simulink model "case3"  (R2024b)
settings: Solver=FixedStepAuto  StartTime=0  StopTime=1  FixedStep=1e-7  RelTol=1e-3
values from neighbouring files (symbols this model uses):
  SG_D_1_D = 0.01056    [IEEE9_case_parameters.m]    (also in case1_parameters.m; case2_parameters.m; case3_parameters.m; case4_parameters.m)
  SG_D_1_EnableSaturation = 0    [IEEE9_case_parameters.m]    (also in case1_parameters.m; case2_parameters.m; case3_parameters.m; case4_parameters.m)
  SG_D_1_f0 = 60    [IEEE9_case_parameters.m]    (also in case1_parameters.m; case2_parameters.m; case3_parameters.m; case4_parameters.m)
  SG_D_1_H = 7.5    [IEEE9_case_parameters.m]    (also in case1_parameters.m; case2_parameters.m; case3_parameters.m; case4_parameters.m)
  SG_D_1_K_A = 20    [IEEE9_case_parameters.m]    (also in case1_parameters.m; case2_parameters.m; case3_parameters.m; case4_parameters.m)
  SG_D_1_K_E = 1.000000e+1    (= 10)    [IEEE9_case_parameters.m]    (also in case1_parameters.m; case2_parameters.m; case3_parameters.m; case4_parameters.m)
  SG_D_1_K_F = 2.363    [IEEE9_case_parameters.m]    (also in case1_parameters.m; case2_parameters.m; case3_parameters.m; case4_parameters.m)
  SG_D_1_K_s = 0.5    [IEEE9_case_parameters.m]    (also in case1_parameters.m = 5; case2_parameters.m = 5; case3_parameters.m = 5; case4_parameters.m = 5)
  SG_D_1_R_a = 0.001088    [IEEE9_case_parameters.m]    (also in case1_parameters.m; case2_parameters.m; case3_parameters.m; case4_parameters.m)
  SG_D_1_S_A = 1    [IEEE9_case_parameters.m]    (also in case1_parameters.m; case2_parameters.m; case3_parameters.m; case4_parameters.m)
  SG_D_1_S_B = 0.103    [IEEE9_case_parameters.m]    (also in case1_parameters.m; case2_parameters.m; case3_parameters.m; case4_parameters.m)
  SG_D_1_S_N = 10.659857    [IEEE9_case_parameters.m]    (also in case1_parameters.m; case2_parameters.m; case3_parameters.m; case4_parameters.m)
  SG_D_1_SpeedPara = 200    [IEEE9_case_parameters.m]    (also in case1_parameters.m; case2_parameters.m; case3_parameters.m; case4_parameters.m)
  SG_D_1_T_0 = 0.720173    [IEEE9_case_parameters.m]    (also in case1_parameters.m = 0.755522; case2_parameters.m = 0.808931; case3_parameters.m = 0.869402; case4_parameters.m = 0.729316)
  SG_D_1_T_1 = 0.3    [IEEE9_case_parameters.m]    (also in case1_parameters.m; case2_parameters.m; case3_parameters.m; case4_parameters.m)
  SG_D_1_T_2 = 0.05    [IEEE9_case_parameters.m]    (also in case1_parameters.m; case2_parameters.m; case3_parameters.m; case4_parameters.m)
  SG_D_1_T_3 = 0.02    [IEEE9_case_parameters.m]    (also in case1_parameters.m; case2_parameters.m; case3_parameters.m; case4_parameters.m)
  SG_D_1_T_4 = 0.005    [IEEE9_case_parameters.m]    (also in case1_parameters.m; case2_parameters.m; case3_parameters.m; case4_parameters.m)
  SG_D_1_T_A = 0.02    [IEEE9_case_parameters.m]    (also in case1_parameters.m; case2_parameters.m; case3_parameters.m; case4_parameters.m)
  SG_D_1_T_dd = 8.000000e+0    (= 8)    [IEEE9_case_parameters.m]    (also in case1_parameters.m; case2_parameters.m; case3_parameters.m; case4_parameters.m)
  SG_D_1_T_ddd = 0.04    [IEEE9_case_parameters.m]    (also in case1_parameters.m; case2_parameters.m; case3_parameters.m; case4_parameters.m)
  SG_D_1_T_E = 0.314    [IEEE9_case_parameters.m]    (also in case1_parameters.m; case2_parameters.m; case3_parameters.m; case4_parameters.m)
  SG_D_1_T_F = 0.35    [IEEE9_case_parameters.m]    (also in case1_parameters.m; case2_parameters.m; case3_parameters.m; case4_parameters.m)
  SG_D_1_T_qd = 0.8    [IEEE9_case_parameters.m]    (also in case1_parameters.m; case2_parameters.m; case3_parameters.m; case4_parameters.m)
  SG_D_1_T_qdd = 0.02    [IEEE9_case_parameters.m]    (also in case1_parameters.m; case2_parameters.m; case3_parameters.m; case4_parameters.m)
  SG_D_1_T_speed = 0.1    [IEEE9_case_parameters.m]    (also in case1_parameters.m = 200; case2_parameters.m = 200; case3_parameters.m = 200; case4_parameters.m = 200)
  SG_D_1_T_w = 0.5    [IEEE9_case_parameters.m]    (also in case1_parameters.m; case2_parameters.m; case3_parameters.m; case4_parameters.m)
  SG_D_1_V_ref = 1.990276    [IEEE9_case_parameters.m]    (also in case1_parameters.m = 2.042296; case2_parameters.m = 2.051388; case3_parameters.m = 2.089584; case4_parameters.m = 2.01845)
  SG_D_1_w_ref = 376.991118    [IEEE9_case_parameters.m]    (also in case1_parameters.m; case2_parameters.m; case3_parameters.m; case4_parameters.m)
  SG_D_1_wb = 6.000000e+1    (= 60)    [IEEE9_case_parameters.m]    (also in case1_parameters.m; case2_parameters.m; case3_parameters.m; case4_parameters.m)
  SG_D_1_x_d = 1.9    [IEEE9_case_parameters.m]    (also in case1_parameters.m; case2_parameters.m; case3_parameters.m; case4_parameters.m)
  SG_D_1_x_dd = 0.302    [IEEE9_case_parameters.m]    (also in case1_parameters.m; case2_parameters.m; case3_parameters.m; case4_parameters.m)
  SG_D_1_x_ddd = 0.204    [IEEE9_case_parameters.m]    (also in case1_parameters.m; case2_parameters.m; case3_parameters.m; case4_parameters.m)
  SG_D_1_x_l = 0.05    [IEEE9_case_parameters.m]    (also in case1_parameters.m; case2_parameters.m; case3_parameters.m; case4_parameters.m)
  SG_D_1_x_q = 1.3    [IEEE9_case_parameters.m]    (also in case1_parameters.m; case2_parameters.m; case3_parameters.m; case4_parameters.m)
  SG_D_1_x_qd = 0.5    [IEEE9_case_parameters.m]    (also in case1_parameters.m; case2_parameters.m; case3_parameters.m; case4_parameters.m)
  SG_D_1_x_qdd = 0.3    [IEEE9_case_parameters.m]    (also in case1_parameters.m; case2_parameters.m; case3_parameters.m; case4_parameters.m)
  SG_D_2_D = 0.02    [IEEE9_case_parameters.m]    (also in case1_parameters.m; case2_parameters.m; case3_parameters.m; case4_parameters.m)
  SG_D_2_EnableSaturation = 0    [IEEE9_case_parameters.m]    (also in case1_parameters.m; case2_parameters.m; case3_parameters.m; case4_parameters.m)
  SG_D_2_f0 = 60    [IEEE9_case_parameters.m]    (also in case1_parameters.m; case2_parameters.m; case3_parameters.m; case4_parameters.m)
  SG_D_2_H = 8.000000e+0    (= 8)    [IEEE9_case_parameters.m]    (also in case1_parameters.m; case2_parameters.m; case3_parameters.m; case4_parameters.m)
  SG_D_2_K_A = 20    [IEEE9_case_parameters.m]    (also in case1_parameters.m; case2_parameters.m; case3_parameters.m; case4_parameters.m)
  SG_D_2_K_E = 1.000000e+1    (= 10)    [IEEE9_case_parameters.m]    (also in case1_parameters.m; case2_parameters.m; case3_parameters.m; case4_parameters.m)
  SG_D_2_K_F = 2.363    [IEEE9_case_parameters.m]    (also in case1_parameters.m; case2_parameters.m; case3_parameters.m; case4_parameters.m)
  SG_D_2_K_s = 0.5    [IEEE9_case_parameters.m]    (also in case1_parameters.m = 4; case2_parameters.m = 4; case3_parameters.m = 4; case4_parameters.m = 4)
  SG_D_2_R_a = 0.001088    [IEEE9_case_parameters.m]    (also in case1_parameters.m; case2_parameters.m; case3_parameters.m; case4_parameters.m)
  SG_D_2_S_A = 1    [IEEE9_case_parameters.m]    (also in case1_parameters.m; case2_parameters.m; case3_parameters.m; case4_parameters.m)
  SG_D_2_S_B = 0.103    [IEEE9_case_parameters.m]    (also in case1_parameters.m; case2_parameters.m; case3_parameters.m; case4_parameters.m)
  SG_D_2_S_N = 10.659857    [IEEE9_case_parameters.m]    (also in case1_parameters.m; case2_parameters.m; case3_parameters.m; case4_parameters.m)
  SG_D_2_SpeedPara = 200    [IEEE9_case_parameters.m]    (also in case1_parameters.m; case2_parameters.m; case3_parameters.m; case4_parameters.m)
  SG_D_2_T_0 = 1.632913    [IEEE9_case_parameters.m]    (also in case1_parameters.m = 1.632925; case2_parameters.m = 1.632915; case3_parameters.m = 1.632914; case4_parameters.m = 1.632927)
  SG_D_2_T_1 = 0.2    [IEEE9_case_parameters.m]    (also in case1_parameters.m; case2_parameters.m; case3_parameters.m; case4_parameters.m)
  SG_D_2_T_2 = 0.05    [IEEE9_case_parameters.m]    (also in case1_parameters.m; case2_parameters.m; case3_parameters.m; case4_parameters.m)
  SG_D_2_T_3 = 0.02    [IEEE9_case_parameters.m]    (also in case1_parameters.m; case2_parameters.m; case3_parameters.m; case4_parameters.m)
  SG_D_2_T_4 = 0.005    [IEEE9_case_parameters.m]    (also in case1_parameters.m; case2_parameters.m; case3_parameters.m; case4_parameters.m)
  SG_D_2_T_A = 0.02    [IEEE9_case_parameters.m]    (also in case1_parameters.m; case2_parameters.m; case3_parameters.m; case4_parameters.m)
  SG_D_2_T_dd = 7.9    [IEEE9_case_parameters.m]    (also in case1_parameters.m; case2_parameters.m; case3_parameters.m; case4_parameters.m)
  SG_D_2_T_ddd = 0.04    [IEEE9_case_parameters.m]    (also in case1_parameters.m; case2_parameters.m; case3_parameters.m; case4_parameters.m)
  SG_D_2_T_E = 0.314    [IEEE9_case_parameters.m]    (also in case1_parameters.m; case2_parameters.m; case3_parameters.m; case4_parameters.m)
  SG_D_2_T_F = 0.35    [IEEE9_case_parameters.m]    (also in case1_parameters.m; case2_parameters.m; case3_parameters.m; case4_parameters.m)
  SG_D_2_T_qd = 0.8    [IEEE9_case_parameters.m]    (also in case1_parameters.m; case2_parameters.m; case3_parameters.m; case4_parameters.m)
  SG_D_2_T_qdd = 0.015    [IEEE9_case_parameters.m]    (also in case1_parameters.m; case2_parameters.m; case3_parameters.m; case4_parameters.m)
  SG_D_2_T_speed = 0.1    [IEEE9_case_parameters.m]    (also in case1_parameters.m = 150; case2_parameters.m = 150; case3_parameters.m = 150; case4_parameters.m = 150)
  SG_D_2_T_w = 0.35    [IEEE9_case_parameters.m]    (also in case1_parameters.m; case2_parameters.m; case3_parameters.m; case4_parameters.m)
  SG_D_2_V_ref = 2.58547    [IEEE9_case_parameters.m]    (also in case1_parameters.m = 2.597896; case2_parameters.m = 2.587136; case3_parameters.m = 2.586042; case4_parameters.m = 2.599679)
  SG_D_2_w_ref = 376.991118    [IEEE9_case_parameters.m]    (also in case1_parameters.m; case2_parameters.m; case3_parameters.m; case4_parameters.m)
  SG_D_2_wb = 6.000000e+1    (= 60)    [IEEE9_case_parameters.m]    (also in case1_parameters.m; case2_parameters.m; case3_parameters.m; case4_parameters.m)
  SG_D_2_x_d = 1.8    [IEEE9_case_parameters.m]    (also in case1_parameters.m; case2_parameters.m; case3_parameters.m; case4_parameters.m)
  SG_D_2_x_dd = 0.302    [IEEE9_case_parameters.m]    (also in case1_parameters.m; case2_parameters.m; case3_parameters.m; case4_parameters.m)
  SG_D_2_x_ddd = 0.204    [IEEE9_case_parameters.m]    (also in case1_parameters.m; case2_parameters.m; case3_parameters.m; case4_parameters.m)
  SG_D_2_x_l = 0.05    [IEEE9_case_parameters.m]    (also in case1_parameters.m; case2_parameters.m; case3_parameters.m; case4_parameters.m)
  SG_D_2_x_q = 1.25    [IEEE9_case_parameters.m]    (also in case1_parameters.m; case2_parameters.m; case3_parameters.m; case4_parameters.m)
  SG_D_2_x_qd = 0.5    [IEEE9_case_parameters.m]    (also in case1_parameters.m; case2_parameters.m; case3_parameters.m; case4_parameters.m)
  SG_D_2_x_qdd = 0.3    [IEEE9_case_parameters.m]    (also in case1_parameters.m; case2_parameters.m; case3_parameters.m; case4_parameters.m)
  SG_D_3_D = 0.02    [IEEE9_case_parameters.m]    (also in case1_parameters.m; case2_parameters.m; case3_parameters.m; case4_parameters.m)
  SG_D_3_EnableSaturation = 0    [IEEE9_case_parameters.m]    (also in case1_parameters.m; case2_parameters.m; case3_parameters.m; case4_parameters.m)
  SG_D_3_f0 = 60    [IEEE9_case_parameters.m]    (also in case1_parameters.m; case2_parameters.m; case3_parameters.m; case4_parameters.m)
  SG_D_3_H = 7.7    [IEEE9_case_parameters.m]    (also in case1_parameters.m; case2_parameters.m; case3_parameters.m; case4_parameters.m)
  SG_D_3_K_A = 20    [IEEE9_case_parameters.m]    (also in case1_parameters.m; case2_parameters.m; case3_parameters.m; case4_parameters.m)
  SG_D_3_K_E = 1.000000e+1    (= 10)    [IEEE9_case_parameters.m]    (also in case1_parameters.m; case2_parameters.m; case3_parameters.m; case4_parameters.m)
  SG_D_3_K_F = 2.363    [IEEE9_case_parameters.m]    (also in case1_parameters.m; case2_parameters.m; case3_parameters.m; case4_parameters.m)
  SG_D_3_K_s = 0.2    [IEEE9_case_parameters.m]    (also in case1_parameters.m = 2; case2_parameters.m = 2; case3_parameters.m = 2; case4_parameters.m = 2)
  SG_D_3_R_a = 0.001088    [IEEE9_case_parameters.m]    (also in case1_parameters.m; case2_parameters.m; case3_parameters.m; case4_parameters.m)
  SG_D_3_S_A = 1    [IEEE9_case_parameters.m]    (also in case1_parameters.m; case2_parameters.m; case3_parameters.m; case4_parameters.m)
  SG_D_3_S_B = 0.103    [IEEE9_case_parameters.m]    (also in case1_parameters.m; case2_parameters.m; case3_parameters.m; case4_parameters.m)
  SG_D_3_S_N = 10.659857    [IEEE9_case_parameters.m]    (also in case1_parameters.m; case2_parameters.m; case3_parameters.m; case4_parameters.m)
  SG_D_3_SpeedPara = 200    [IEEE9_case_parameters.m]    (also in case1_parameters.m; case2_parameters.m; case3_parameters.m; case4_parameters.m)
  SG_D_3_T_0 = 0.850788    [IEEE9_case_parameters.m]    (also in case1_parameters.m = 0.850786; case2_parameters.m = 0.850787; case3_parameters.m; case4_parameters.m = 0.850786)
  SG_D_3_T_1 = 0.2    [IEEE9_case_parameters.m]    (also in case1_parameters.m; case2_parameters.m; case3_parameters.m; case4_parameters.m)
  SG_D_3_T_2 = 0.05    [IEEE9_case_parameters.m]    (also in case1_parameters.m; case2_parameters.m; case3_parameters.m; case4_parameters.m)
  SG_D_3_T_3 = 0.02    [IEEE9_case_parameters.m]    (also in case1_parameters.m; case2_parameters.m; case3_parameters.m; case4_parameters.m)
  SG_D_3_T_4 = 0.005    [IEEE9_case_parameters.m]    (also in case1_parameters.m; case2_parameters.m; case3_parameters.m; case4_parameters.m)
  SG_D_3_T_A = 0.02    [IEEE9_case_parameters.m]    (also in case1_parameters.m; case2_parameters.m; case3_parameters.m; case4_parameters.m)
  SG_D_3_T_dd = 8.1    [IEEE9_case_parameters.m]    (also in case1_parameters.m; case2_parameters.m; case3_parameters.m; case4_parameters.m)
  SG_D_3_T_ddd = 0.04    [IEEE9_case_parameters.m]    (also in case1_parameters.m; case2_parameters.m; case3_parameters.m; case4_parameters.m)
  SG_D_3_T_E = 0.314    [IEEE9_case_parameters.m]    (also in case1_parameters.m; case2_parameters.m; case3_parameters.m; case4_parameters.m)
  SG_D_3_T_F = 0.35    [IEEE9_case_parameters.m]    (also in case1_parameters.m; case2_parameters.m; case3_parameters.m; case4_parameters.m)
  SG_D_3_T_qd = 0.8    [IEEE9_case_parameters.m]    (also in case1_parameters.m; case2_parameters.m; case3_parameters.m; case4_parameters.m)
  SG_D_3_T_qdd = 0.015    [IEEE9_case_parameters.m]    (also in case1_parameters.m; case2_parameters.m; case3_parameters.m; case4_parameters.m)
  SG_D_3_T_speed = 0.1    [IEEE9_case_parameters.m]    (also in case1_parameters.m = 180; case2_parameters.m = 180; case3_parameters.m = 180; case4_parameters.m = 180)
  SG_D_3_T_w = 0.4    [IEEE9_case_parameters.m]    (also in case1_parameters.m; case2_parameters.m; case3_parameters.m; case4_parameters.m)
  SG_D_3_V_ref = 1.892727    [IEEE9_case_parameters.m]    (also in case1_parameters.m = 1.906439; case2_parameters.m = 1.895535; case3_parameters.m = 1.892105; case4_parameters.m = 1.906598)
  SG_D_3_w_ref = 376.991118    [IEEE9_case_parameters.m]    (also in case1_parameters.m; case2_parameters.m; case3_parameters.m; case4_parameters.m)
  SG_D_3_wb = 6.000000e+1    (= 60)    [IEEE9_case_parameters.m]    (also in case1_parameters.m; case2_parameters.m; case3_parameters.m; case4_parameters.m)
  SG_D_3_x_d = 1.85    [IEEE9_case_parameters.m]    (also in case1_parameters.m; case2_parameters.m; case3_parameters.m; case4_parameters.m)
  SG_D_3_x_dd = 0.302    [IEEE9_case_parameters.m]    (also in case1_parameters.m; case2_parameters.m; case3_parameters.m; case4_parameters.m)
  SG_D_3_x_ddd = 0.204    [IEEE9_case_parameters.m]    (also in case1_parameters.m; case2_parameters.m; case3_parameters.m; case4_parameters.m)
  SG_D_3_x_l = 0.05    [IEEE9_case_parameters.m]    (also in case1_parameters.m; case2_parameters.m; case3_parameters.m; case4_parameters.m)
  SG_D_3_x_q = 1.2    [IEEE9_case_parameters.m]    (also in case1_parameters.m; case2_parameters.m; case3_parameters.m; case4_parameters.m)
  SG_D_3_x_qd = 0.5    [IEEE9_case_parameters.m]    (also in case1_parameters.m; case2_parameters.m; case3_parameters.m; case4_parameters.m)
  SG_D_3_x_qdd = 0.3    [IEEE9_case_parameters.m]    (also in case1_parameters.m; case2_parameters.m; case3_parameters.m; case4_parameters.m)
(part 6 of 12)

== system case3/SG_D_1/d_psi_kq_SG_D_1_block ==
  note: d_psi_kq_SG_D_1 in case3
      | $-\frac{\psi _{\mathrm{gq},\mathrm{SG},D,1}+\psi _{\mathrm{kq},\mathrm{SG},D,1}+\frac{\left(x_{l}-x_{\mathrm{qd}}\right)\,\left(\psi _{q,\mathrm{SG},D,1}+\frac{\psi _{\mathrm{gq},\mathrm{SG},D,1}\,\left(x_{l}-x_{\mathrm{qdd}}\right)}{x_{l}-x_{\mathrm{qd}}}+\frac{\psi _{\mathrm{kq},\mathrm{SG},D,1}\,\left(x_{\mathrm{qd}}-x_{\mathrm{qdd}}\right)}{x_{l}-x_{\mathrm{qd}}}\right)}{x_{\mathrm{qdd}}}}{T_{\mathrm{qdd}}}$
      | Automatically generated on 2025-10-31 18:59:02 .
  State_psi_gq_SG_D_1_92ffe : Inport
  State_psi_kq_SG_D_1_e445d : Inport  Port=2
  State_psi_gq_SG_D_1_b227a : Inport  Port=3
  State_psi_kq_SG_D_1_06d41 : Inport  Port=4
  State_psi_q_SG_D_1_463f3 : Inport  Port=5
  Add_10dd6 : Sum
  Add_2ce7c : Sum
  Add_45348 : Sum
  Add_70ba0 : Sum
  Add_be2ea : Sum
  Add_ee481 : Sum
  Constant_-1_16d72 : Constant  Value=-1
  Constant_-1_591cb : Constant  Value=-1
  Constant_-1_c1b7c : Constant  Value=-1
  Constant_-1_e0c66 : Constant  Value=-1
  Constant_-1_e7514 : Constant  Value=-1
  Constant_T_qdd_225d4 : Constant  Value=T_qdd
  Constant_x_l_29880 : Constant  Value=x_l
  Constant_x_l_33df5 : Constant  Value=x_l
  Constant_x_l_9cbc8 : Constant  Value=x_l
  Constant_x_l_abab9 : Constant  Value=x_l
  Constant_x_qd_144ef : Constant  Value=x_qd
  Constant_x_qd_60deb : Constant  Value=x_qd
  Constant_x_qd_a807f : Constant  Value=x_qd
  Constant_x_qd_dc41b : Constant  Value=x_qd
  Constant_x_qdd_4bbb9 : Constant  Value=x_qdd
  Constant_x_qdd_9fa02 : Constant  Value=x_qdd
  Constant_x_qdd_d5cad : Constant  Value=x_qdd
  Divide_89ec1 : Product  Inputs=*/
  Divide_a94b2 : Product  Inputs=*/
  Divide_bf1a4 : Product  Inputs=*/
  Divide_ee185 : Product  Inputs=*/
  Product_0063f : Product
  Product_22864 : Product
  Product_2aeff : Product
  Product_365aa : Product
  Product_85a20 : Product
  Product_a1ae8 : Product
  Product_a8586 : Product
  Product_e1897 : Product
  Subtract_1d41a : Sum  Inputs=+-
  Subtract_47a1e : Sum  Inputs=+-
  Subtract_7e7d4 : Sum  Inputs=+-
  Blockout_d_psi_kq_SG_D_1_a4a4a : Outport
  wires:
  Product_a8586/1 -> Add_45348/1
  Constant_-1_e7514/1 -> Product_a8586/1
  Constant_x_l_9cbc8/1 -> Product_a8586/2
  Constant_x_qdd_4bbb9/1 -> Add_45348/2
  Constant_-1_591cb/1 -> Product_365aa/1
  Constant_x_qd_144ef/1 -> Subtract_47a1e/1
  Constant_x_qd_60deb/1 -> Add_70ba0/2
  Constant_-1_e0c66/1 -> Product_2aeff/1
  Constant_x_l_33df5/1 -> Product_365aa/2
  Constant_x_qdd_d5cad/1 -> Subtract_47a1e/2
  Constant_x_qd_a807f/1 -> Add_ee481/2
  Constant_x_l_29880/1 -> Product_2aeff/2
  Subtract_1d41a/1 -> Add_be2ea/1
  Product_0063f/1 -> Subtract_1d41a/1
  State_psi_gq_SG_D_1_b227a/1 -> Product_22864/1
  Add_45348/1 -> Product_22864/2
  Product_2aeff/1 -> Add_10dd6/1
  Constant_x_qd_dc41b/1 -> Add_10dd6/2
  State_psi_kq_SG_D_1_06d41/1 -> Product_85a20/1
  Product_365aa/1 -> Add_ee481/1
  Subtract_47a1e/1 -> Product_85a20/2
  Product_22864/1 -> Divide_ee185/1
  Add_10dd6/1 -> Divide_ee185/2
  Product_85a20/1 -> Divide_bf1a4/1
  Add_ee481/1 -> Divide_bf1a4/2
  Constant_-1_16d72/1 -> Product_e1897/1
  Constant_x_l_abab9/1 -> Product_e1897/2
  Divide_ee185/1 -> Subtract_7e7d4/1
  Divide_bf1a4/1 -> Subtract_7e7d4/2
  Product_e1897/1 -> Add_70ba0/1
  Add_2ce7c/1 -> Product_a1ae8/2
  Subtract_7e7d4/1 -> Add_2ce7c/1
  State_psi_q_SG_D_1_463f3/1 -> Add_2ce7c/2
  Constant_-1_c1b7c/1 -> Product_0063f/1
  State_psi_gq_SG_D_1_92ffe/1 -> Product_0063f/2
  Divide_89ec1/1 -> Add_be2ea/2
  Product_a1ae8/1 -> Divide_89ec1/1
  Add_70ba0/1 -> Product_a1ae8/1
  State_psi_kq_SG_D_1_e445d/1 -> Subtract_1d41a/2
  Constant_x_qdd_9fa02/1 -> Divide_89ec1/2
  Add_be2ea/1 -> Divide_a94b2/1
  Constant_T_qdd_225d4/1 -> Divide_a94b2/2
  Divide_a94b2/1 -> Blockout_d_psi_kq_SG_D_1_a4a4a/1

== system case3/SG_D_1/d_psi_q_SG_D_1_block ==
  note: d_psi_q_SG_D_1 in case3
      | $2\,\pi \,f_{0}\,\left(v_{d,\mathrm{SG},D,1}\,\cos\left(\theta _{\mathrm{SG},D,1}\right)+v_{q,\mathrm{SG},D,1}\,\sin\left(\theta _{\mathrm{SG},D,1}\right)-\frac{R_{a}\,\left(\psi _{q,\mathrm{SG},D,1}+\frac{\psi _{\mathrm{gq},\mathrm{SG},D,1}\,\left(x_{l}-x_{\mathrm{qdd}}\right)}{x_{l}-x_{\mathrm{qd}}}+\frac{\psi _{\mathrm{kq},\mathrm{SG},D,1}\,\left(x_{\mathrm{qd}}-x_{\mathrm{qdd}}\right)}{x_{l}-x_{\mathrm{qd}}}\right)}{x_{\mathrm{qdd}}}-\frac{\psi _{d,\mathrm{SG},D,1}\,w_{\mathrm{SG},D,1}}{2\,f_{0}\,\pi }\right)$
      | Automatically generated on 2025-10-31 18:58:44 .
  State_psi_gq_SG_D_1_d9645 : Inport
  State_psi_kq_SG_D_1_5e11c : Inport  Port=2
  State_psi_q_SG_D_1_8b0a5 : Inport  Port=3
  Input_v_d_SG_D_1_19fdc : Inport  Port=4
  State_theta_SG_D_1_3237f : Inport  Port=5
  Input_v_q_SG_D_1_e60b4 : Inport  Port=6
  State_theta_SG_D_1_9067a : Inport  Port=7
  State_psi_d_SG_D_1_31d3d : Inport  Port=8
  State_w_SG_D_1_cf84f : Inport  Port=9
  Add_253c8 : Sum
  Add_34d81 : Sum
  Add_5178e : Sum
  Add_b73e6 : Sum
  Add_f023d : Sum
  Constant_-1_05677 : Constant  Value=-1
  Constant_-1_3fa46 : Constant  Value=-1
  Constant_-1_c9ea3 : Constant  Value=-1
  Constant_-2.0_60d0e : Constant  Value=-2.0
  Constant_2.0_df2a4 : Constant  Value=2.0
  Constant_R_a_eca46 : Constant  Value=R_a
  Constant_f0_48930 : Constant  Value=f0
  Constant_f0_adbfb : Constant  Value=f0
  Constant_pi_2c23b : Constant  Value=pi
  Constant_pi_82143 : Constant  Value=pi
  Constant_x_l_6866e : Constant  Value=x_l
  Constant_x_l_774e0 : Constant  Value=x_l
  Constant_x_l_b2b5d : Constant  Value=x_l
  Constant_x_qd_0c42a : Constant  Value=x_qd
  Constant_x_qd_28a34 : Constant  Value=x_qd
  Constant_x_qd_d1a4b : Constant  Value=x_qd
  Constant_x_qdd_45d63 : Constant  Value=x_qdd
  Constant_x_qdd_a6763 : Constant  Value=x_qdd
  Constant_x_qdd_ac017 : Constant  Value=x_qdd
  Divide_0b9a2 : Product  Inputs=*/
  Divide_629b9 : Product  Inputs=*/
  Divide_747e5 : Product  Inputs=*/
  Divide_9e6e8 : Product  Inputs=*/
  MathFunc_cos_ef02a : Trigonometry  Operator=cos
  MathFunc_sin_6bc4f : Trigonometry
  Product_044b2 : Product
  Product_15984 : Product
  Product_19e84 : Product
  Product_3860a : Product
  Product_6486c : Product
  Product_67e3c : Product
  Product_6c70c : Product
  Product_79b02 : Product
  Product_8bf86 : Product
  Product_91a21 : Product
  Product_9d3a2 : Product
  Product_ad3ba : Product
  Product_ba60d : Product
  Product_c079b : Product
  Subtract_09d9d : Sum  Inputs=+-
  Subtract_0f2d7 : Sum  Inputs=+-
  Subtract_13675 : Sum  Inputs=+-
  Subtract_f028b : Sum  Inputs=+-
  Blockout_d_psi_q_SG_D_1_513bd : Outport
  wires:
  Divide_0b9a2/1 -> Subtract_13675/1
  Product_9d3a2/1 -> Add_253c8/1
  Constant_x_l_b2b5d/1 -> Product_9d3a2/2
  Constant_-1_05677/1 -> Product_9d3a2/1
  Constant_x_qdd_45d63/1 -> Add_253c8/2
  Constant_x_l_774e0/1 -> Product_ba60d/2
  Constant_-1_c9ea3/1 -> Product_ba60d/1
  Constant_x_l_6866e/1 -> Product_67e3c/2
  Constant_x_qdd_ac017/1 -> Subtract_09d9d/2
  State_psi_kq_SG_D_1_5e11c/1 -> Product_6486c/1
  Constant_-1_3fa46/1 -> Product_67e3c/1
  Constant_x_qd_0c42a/1 -> Subtract_09d9d/1
  State_psi_gq_SG_D_1_d9645/1 -> Product_3860a/1
  Product_15984/1 -> Blockout_d_psi_q_SG_D_1_513bd/1
  Subtract_13675/1 -> Add_34d81/1
  Product_3860a/1 -> Divide_0b9a2/1
  Add_253c8/1 -> Product_3860a/2
  Divide_9e6e8/1 -> Subtract_13675/2
  Product_ba60d/1 -> Add_5178e/1
  Constant_x_qd_28a34/1 -> Add_5178e/2
  Constant_-2.0_60d0e/1 -> Product_91a21/1
  Product_6486c/1 -> Divide_9e6e8/1
  Product_67e3c/1 -> Add_f023d/1
  Subtract_09d9d/1 -> Product_6486c/2
  Constant_x_qd_d1a4b/1 -> Add_f023d/2
  Add_5178e/1 -> Divide_0b9a2/2
  Add_f023d/1 -> Divide_9e6e8/2
  Constant_f0_48930/1 -> Product_ad3ba/2
  State_psi_q_SG_D_1_8b0a5/1 -> Add_34d81/2
  Product_19e84/1 -> Product_c079b/1
  Constant_R_a_eca46/1 -> Product_6c70c/1
  Product_c079b/1 -> Divide_747e5/2
  Product_6c70c/1 -> Divide_629b9/1
  Add_34d81/1 -> Product_6c70c/2
  State_theta_SG_D_1_3237f/1 -> MathFunc_cos_ef02a/1
  Input_v_d_SG_D_1_19fdc/1 -> Product_8bf86/1
  Constant_x_qdd_a6763/1 -> Divide_629b9/2
  MathFunc_cos_ef02a/1 -> Product_8bf86/2
  State_theta_SG_D_1_9067a/1 -> MathFunc_sin_6bc4f/1
  Divide_629b9/1 -> Subtract_0f2d7/1
  Constant_2.0_df2a4/1 -> Product_19e84/1
  State_w_SG_D_1_cf84f/1 -> Product_79b02/2
  Constant_pi_82143/1 -> Product_19e84/2
  Subtract_f028b/1 -> Add_b73e6/1
  Product_8bf86/1 -> Subtract_0f2d7/2
  Divide_747e5/1 -> Add_b73e6/2
  Input_v_q_SG_D_1_e60b4/1 -> Product_044b2/1
  MathFunc_sin_6bc4f/1 -> Product_044b2/2
  Product_044b2/1 -> Subtract_f028b/2
  State_psi_d_SG_D_1_31d3d/1 -> Product_79b02/1
  Constant_f0_adbfb/1 -> Product_c079b/2
  Constant_pi_2c23b/1 -> Product_91a21/2
  Subtract_0f2d7/1 -> Subtract_f028b/1
  Product_79b02/1 -> Divide_747e5/1
  Product_91a21/1 -> Product_ad3ba/1
  Product_ad3ba/1 -> Product_15984/1
  Add_b73e6/1 -> Product_15984/2

== system case3/SG_D_1/d_theta_SG_D_1_block ==
  note: d_theta_SG_D_1 in case3
      | $w_{\mathrm{SG},D,1}-2\,\pi \,f_{0}$
      | Automatically generated on 2025-10-31 18:59:10 .
  State_w_SG_D_1_fb02a : Inport
  Add_76eb3 : Sum
  Constant_-2.0_a4ed5 : Constant  Value=-2.0
  Constant_f0_72e60 : Constant  Value=f0
  Constant_pi_ad9ad : Constant  Value=pi
  Product_49826 : Product
  Product_bc9e7 : Product
  Blockout_d_theta_SG_D_1_4a614 : Outport
  wires:
  State_w_SG_D_1_fb02a/1 -> Add_76eb3/2
  Constant_-2.0_a4ed5/1 -> Product_49826/1
  Constant_f0_72e60/1 -> Product_bc9e7/2
  Constant_pi_ad9ad/1 -> Product_49826/2
  Product_bc9e7/1 -> Add_76eb3/1
  Product_49826/1 -> Product_bc9e7/1
  Add_76eb3/1 -> Blockout_d_theta_SG_D_1_4a614/1

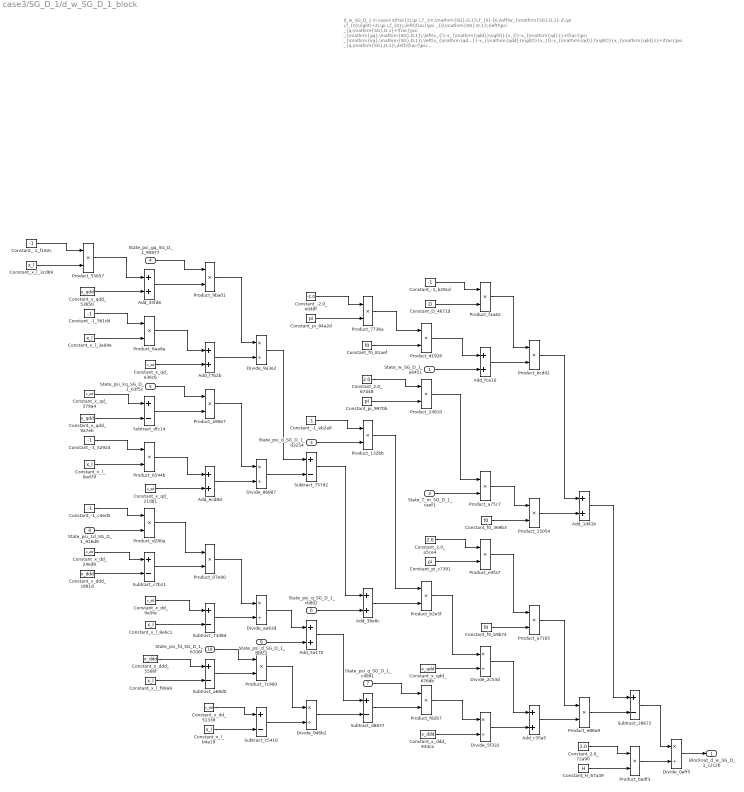
== system case3/SG_D_1/d_w_SG_D_1_block ==
  note: d_w_SG_D_1 in case3
      | $\frac{2\,\pi \,T_{m,\mathrm{SG},D,1}\,f_{0}-D\,\left(w_{\mathrm{SG},D,1}-2\,\pi \,f_{0}\right)+2\,\pi \,f_{0}\,\left(\frac{\psi _{d,\mathrm{SG},D,1}\,\left(\psi _{q,\mathrm{SG},D,1}+\frac{\psi _{\mathrm{gq},\mathrm{SG},D,1}\,\left(x_{l}-x_{\mathrm{qdd}}\right)}{x_{l}-x_{\mathrm{qd}}}+\frac{\psi _{\mathrm{kq},\mathrm{SG},D,1}\,\left(x_{\mathrm{qd}}-x_{\mathrm{qdd}}\right)}{x_{l}-x_{\mathrm{qd}}}\right)}{x_{\mathrm{qdd}}}+\frac{\psi _{q,\mathrm{SG},D,1}\,\left(\frac{\psi _{\mathrm{1d},\mathrm{SG},D,1}\,\left(x_{\mathrm{dd}}-x_{\mathrm{ddd}}\right)}{x_{\mathrm{dd}}-x_{l}}-\psi _{d,\mathrm{SG},D,1}+\frac{\psi _{\mathrm{fd},\mathrm{SG},D,1}\,\left(x_{\mathrm{ddd}}-x_{l}\right)}{x_{\mathrm{dd}}-x_{l}}\right)}{x_{\mathrm{ddd}}}\right)}{2\,H}$
      | Automatically generated on 2025-10-31 18:59:08 .
  State_w_SG_D_1_a6451 : Inport
  State_T_m_SG_D_1_caef1 : Inport  Port=2
  State_psi_d_SG_D_1_d3254 : Inport  Port=3
  State_psi_gq_SG_D_1_95977 : Inport  Port=4
  State_psi_kq_SG_D_1_63f5c : Inport  Port=5
  State_psi_q_SG_D_1_cb802 : Inport  Port=6
  State_psi_q_SG_D_1_c4891 : Inport  Port=7
  State_psi_1d_SG_D_1_916d9 : Inport  Port=8
  State_psi_d_SG_D_1_bbfc2 : Inport  Port=9
  State_psi_fd_SG_D_1_6708f : Inport  Port=10
  Add_1d41b : Sum
  Add_35fd6 : Sum
  Add_38e8c : Sum
  Add_5a170 : Sum
  Add_c35a5 : Sum
  Add_ecd8d : Sum
  Add_f7b2b : Sum
  Add_fce10 : Sum
  Constant_-1_5292d : Constant  Value=-1
  Constant_-1_561d4 : Constant  Value=-1
  Constant_-1_b29cd : Constant  Value=-1
  Constant_-1_c4ed5 : Constant  Value=-1
  Constant_-1_eb2a8 : Constant  Value=-1
  Constant_-1_f182c : Constant  Value=-1
  Constant_-2.0_e048f : Constant  Value=-2.0
  Constant_2.0_67448 : Constant  Value=2.0
  Constant_2.0_72a90 : Constant  Value=2.0
  Constant_2.0_a5ce4 : Constant  Value=2.0
  Constant_D_4671d : Constant  Value=D
  Constant_H_67a49 : Constant  Value=H
  Constant_f0_369b3 : Constant  Value=f0
  Constant_f0_81aef : Constant  Value=f0
  Constant_f0_b9b74 : Constant  Value=f0
  Constant_pi_84a2d : Constant  Value=pi
  Constant_pi_9970b : Constant  Value=pi
  Constant_pi_c7391 : Constant  Value=pi
  Constant_x_dd_24ed8 : Constant  Value=x_dd
  Constant_x_dd_5133d : Constant  Value=x_dd
  Constant_x_dd_9e5fe : Constant  Value=x_dd
  Constant_x_ddd_5566f : Constant  Value=x_ddd
  Constant_x_ddd_934ca : Constant  Value=x_ddd
  Constant_x_ddd_c891d : Constant  Value=x_ddd
  Constant_x_l_0ed79 : Constant  Value=x_l
  Constant_x_l_3a04e : Constant  Value=x_l
  Constant_x_l_3cd69 : Constant  Value=x_l
  Constant_x_l_8e6c1 : Constant  Value=x_l
  Constant_x_l_b4a19 : Constant  Value=x_l
  Constant_x_l_f99a9 : Constant  Value=x_l
  Constant_x_qd_21d81 : Constant  Value=x_qd
  Constant_x_qd_379a4 : Constant  Value=x_qd
  Constant_x_qd_e36c6 : Constant  Value=x_qd
  Constant_x_qdd_53650 : Constant  Value=x_qdd
  Constant_x_qdd_676db : Constant  Value=x_qdd
  Constant_x_qdd_9a7eb : Constant  Value=x_qdd
  Divide_0aff5 : Product  Inputs=*/
  Divide_2c53d : Product  Inputs=*/
  Divide_5f332 : Product  Inputs=*/
  Divide_86887 : Product  Inputs=*/
  Divide_946b2 : Product  Inputs=*/
  Divide_9a3e2 : Product  Inputs=*/
  Divide_aa63d : Product  Inputs=*/
  Product_07e90 : Product
  Product_132bb : Product
  Product_15054 : Product
  Product_24810 : Product
  Product_55657 : Product
  Product_6544b : Product
  Product_6adf3 : Product
  Product_6ea8a : Product
  Product_7736a : Product
  Product_7c900 : Product
  Product_9ba01 : Product
  Product_a71b5 : Product
  Product_a75c7 : Product
  Product_a90e7 : Product
  Product_b2e5f : Product
  Product_bcd42 : Product
  Product_d1926 : Product
  Product_d280a : Product
  Product_e3fa7 : Product
  Product_e88a9 : Product
  Product_f82b7 : Product
  Product_faa62 : Product
  Subtract_28672 : Sum  Inputs=+-
  Subtract_73d8d : Sum  Inputs=+-
  Subtract_757d2 : Sum  Inputs=+-
  Subtract_a68d0 : Sum  Inputs=+-
  Subtract_c5410 : Sum  Inputs=+-
  Subtract_c7b11 : Sum  Inputs=+-
  Subtract_d8837 : Sum  Inputs=+-
  Subtract_dfc14 : Sum  Inputs=+-
  Blockout_d_w_SG_D_1_c2c2b : Outport
  wires:
  Product_d1926/1 -> Add_fce10/1
  Constant_-1_f182c/1 -> Product_55657/1
  Constant_pi_9970b/1 -> Product_24810/2
  Constant_x_qdd_53650/1 -> Add_35fd6/2
  Constant_x_l_3cd69/1 -> Product_55657/2
  Product_55657/1 -> Add_35fd6/1
  Constant_x_qd_379a4/1 -> Subtract_dfc14/1
  Constant_-1_561d4/1 -> Product_6ea8a/1
  Product_7736a/1 -> Product_d1926/1
  Constant_x_qdd_9a7eb/1 -> Subtract_dfc14/2
  State_psi_q_SG_D_1_c4891/1 -> Product_f82b7/1
  Constant_x_l_3a04e/1 -> Product_6ea8a/2
  Constant_-1_5292d/1 -> Product_6544b/1
  Constant_x_l_0ed79/1 -> Product_6544b/2
  Constant_-1_c4ed5/1 -> Product_d280a/1
  Product_6ea8a/1 -> Add_f7b2b/1
  State_psi_1d_SG_D_1_916d9/1 -> Product_d280a/2
  Constant_x_dd_24ed8/1 -> Subtract_c7b11/1
  Subtract_dfc14/1 -> Product_a90e7/2
  Constant_x_ddd_c891d/1 -> Subtract_c7b11/2
  State_psi_gq_SG_D_1_95977/1 -> Product_9ba01/1
  Product_132bb/1 -> Product_b2e5f/1
  Add_35fd6/1 -> Product_9ba01/2
  Constant_x_qd_e36c6/1 -> Add_f7b2b/2
  State_psi_kq_SG_D_1_63f5c/1 -> Product_a90e7/1
  Constant_f0_81aef/1 -> Product_d1926/2
  Product_6544b/1 -> Add_ecd8d/1
  Constant_x_dd_9e5fe/1 -> Subtract_73d8d/1
  Constant_x_qd_21d81/1 -> Add_ecd8d/2
  Product_d280a/1 -> Product_07e90/1
  Subtract_c7b11/1 -> Product_07e90/2
  Constant_x_l_8e6c1/1 -> Subtract_73d8d/2
  Constant_x_ddd_5566f/1 -> Subtract_a68d0/1
  Constant_x_l_f99a9/1 -> Subtract_a68d0/2
  State_w_SG_D_1_a6451/1 -> Add_fce10/2
  Divide_2c53d/1 -> Add_c35a5/1
  Constant_-1_b29cd/1 -> Product_faa62/1
  Product_9ba01/1 -> Divide_9a3e2/1
  Add_fce10/1 -> Product_bcd42/2
  Divide_9a3e2/1 -> Subtract_757d2/1
  Add_f7b2b/1 -> Divide_9a3e2/2
  Constant_pi_84a2d/1 -> Product_7736a/2
  Product_a90e7/1 -> Divide_86887/1
  Add_ecd8d/1 -> Divide_86887/2
  Product_07e90/1 -> Divide_aa63d/1
  Divide_aa63d/1 -> Add_5a170/1
  Subtract_73d8d/1 -> Divide_aa63d/2
  State_psi_fd_SG_D_1_6708f/1 -> Product_7c900/1
  Subtract_a68d0/1 -> Product_7c900/2
  Constant_x_dd_5133d/1 -> Subtract_c5410/1
  Constant_x_l_b4a19/1 -> Subtract_c5410/2
  Divide_86887/1 -> Subtract_757d2/2
  Constant_2.0_67448/1 -> Product_24810/1
  State_psi_d_SG_D_1_bbfc2/1 -> Add_5a170/2
  Product_7c900/1 -> Divide_946b2/1
  Subtract_c5410/1 -> Divide_946b2/2
  Constant_-2.0_e048f/1 -> Product_7736a/1
  Constant_-1_eb2a8/1 -> Product_132bb/1
  State_psi_d_SG_D_1_d3254/1 -> Product_132bb/2
  Subtract_757d2/1 -> Add_38e8c/1
  Subtract_d8837/1 -> Product_f82b7/2
  State_psi_q_SG_D_1_cb802/1 -> Add_38e8c/2
  Add_5a170/1 -> Subtract_d8837/1
  Divide_946b2/1 -> Subtract_d8837/2
  Add_38e8c/1 -> Product_b2e5f/2
  Constant_D_4671d/1 -> Product_faa62/2
  Product_24810/1 -> Product_a75c7/1
  State_T_m_SG_D_1_caef1/1 -> Product_a75c7/2
  Constant_2.0_a5ce4/1 -> Product_e3fa7/1
  Constant_pi_c7391/1 -> Product_e3fa7/2
  Product_b2e5f/1 -> Divide_2c53d/1
  Constant_x_qdd_676db/1 -> Divide_2c53d/2
  Product_f82b7/1 -> Divide_5f332/1
  Constant_x_ddd_934ca/1 -> Divide_5f332/2
  Product_faa62/1 -> Product_bcd42/1
  Product_a75c7/1 -> Product_15054/1
  Constant_f0_369b3/1 -> Product_15054/2
  Product_e3fa7/1 -> Product_a71b5/1
  Constant_f0_b9b74/1 -> Product_a71b5/2
  Divide_5f332/1 -> Add_c35a5/2
  Product_bcd42/1 -> Add_1d41b/1
  Product_15054/1 -> Add_1d41b/2
  Product_a71b5/1 -> Product_e88a9/1
  Add_c35a5/1 -> Product_e88a9/2
  Add_1d41b/1 -> Subtract_28672/1
  Product_e88a9/1 -> Subtract_28672/2
  Constant_2.0_72a90/1 -> Product_6adf3/1
  Constant_H_67a49/1 -> Product_6adf3/2
  Subtract_28672/1 -> Divide_0aff5/1
  Product_6adf3/1 -> Divide_0aff5/2
  Divide_0aff5/1 -> Blockout_d_w_SG_D_1_c2c2b/1

== system case3/SG_D_1/i_d_SG_D_1_block ==
  note: i_d_SG_D_1 in case3
      | $\frac{\sin\left(\theta _{\mathrm{SG},D,1}\right)\,\left(\frac{\psi _{\mathrm{1d},\mathrm{SG},D,1}\,\left(x_{\mathrm{dd}}-x_{\mathrm{ddd}}\right)}{x_{\mathrm{dd}}-x_{l}}-\psi _{d,\mathrm{SG},D,1}+\frac{\psi _{\mathrm{fd},\mathrm{SG},D,1}\,\left(x_{\mathrm{ddd}}-x_{l}\right)}{x_{\mathrm{dd}}-x_{l}}\right)}{x_{\mathrm{ddd}}}-\frac{\cos\left(\theta _{\mathrm{SG},D,1}\right)\,\left(\psi _{q,\mathrm{SG},D,1}+\frac{\psi _{\mathrm{gq},\mathrm{SG},D,1}\,\left(x_{l}-x_{\mathrm{qdd}}\right)}{x_{l}-x_{\mathrm{qd}}}+\frac{\psi _{\mathrm{kq},\mathrm{SG},D,1}\,\left(x_{\mathrm{qd}}-x_{\mathrm{qdd}}\right)}{x_{l}-x_{\mathrm{qd}}}\right)}{x_{\mathrm{qdd}}}$
      | Automatically generated on 2025-10-31 18:59:30 .
  State_psi_gq_SG_D_1_06924 : Inport
  State_psi_kq_SG_D_1_04692 : Inport  Port=2
  State_psi_q_SG_D_1_1a988 : Inport  Port=3
  State_theta_SG_D_1_ace1c : Inport  Port=4
  State_psi_1d_SG_D_1_017fc : Inport  Port=5
  State_psi_d_SG_D_1_ee150 : Inport  Port=6
  State_psi_fd_SG_D_1_d596f : Inport  Port=7
  State_theta_SG_D_1_7475d : Inport  Port=8
  Add_2610a : Sum
  Add_2e8b6 : Sum
  Add_6e688 : Sum
  Add_9e60c : Sum
  Add_b559d : Sum
  Constant_-1_005d7 : Constant  Value=-1
  Constant_-1_0dfb2 : Constant  Value=-1
  Constant_-1_51d10 : Constant  Value=-1
  Constant_-1_b9eea : Constant  Value=-1
  Constant_-1_e05e3 : Constant  Value=-1
  Constant_x_dd_8242f : Constant  Value=x_dd
  Constant_x_dd_b3416 : Constant  Value=x_dd
  Constant_x_dd_bb0c8 : Constant  Value=x_dd
  Constant_x_ddd_2a6be : Constant  Value=x_ddd
  Constant_x_ddd_39085 : Constant  Value=x_ddd
  Constant_x_ddd_e1583 : Constant  Value=x_ddd
  Constant_x_l_26c6b : Constant  Value=x_l
  Constant_x_l_b74c1 : Constant  Value=x_l
  Constant_x_l_c7e57 : Constant  Value=x_l
  Constant_x_l_cb232 : Constant  Value=x_l
  Constant_x_l_cd88d : Constant  Value=x_l
  Constant_x_l_ff016 : Constant  Value=x_l
  Constant_x_qd_64ab0 : Constant  Value=x_qd
  Constant_x_qd_b849d : Constant  Value=x_qd
  Constant_x_qd_e0d58 : Constant  Value=x_qd
  Constant_x_qdd_134fa : Constant  Value=x_qdd
  Constant_x_qdd_9bdcd : Constant  Value=x_qdd
  Constant_x_qdd_f3715 : Constant  Value=x_qdd
  Divide_15d94 : Product  Inputs=*/
  Divide_1dc21 : Product  Inputs=*/
  Divide_4b9cf : Product  Inputs=*/
  Divide_7b0e4 : Product  Inputs=*/
  Divide_aec55 : Product  Inputs=*/
  Divide_f4998 : Product  Inputs=*/
  MathFunc_cos_2d020 : Trigonometry  Operator=cos
  MathFunc_sin_75e4b : Trigonometry
  Product_07601 : Product
  Product_2fce4 : Product
  Product_30dc6 : Product
  Product_4bd24 : Product
  Product_8023f : Product
  Product_8793c : Product
  Product_8e0a1 : Product
  Product_9d8c5 : Product
  Product_b0550 : Product
  Product_b336d : Product
  Product_e93c7 : Product
  Subtract_20919 : Sum  Inputs=+-
  Subtract_322c6 : Sum  Inputs=+-
  Subtract_45595 : Sum  Inputs=+-
  Subtract_92451 : Sum  Inputs=+-
  Subtract_c67a9 : Sum  Inputs=+-
  Subtract_cd319 : Sum  Inputs=+-
  Subtract_d3172 : Sum  Inputs=+-
  Subtract_eb230 : Sum  Inputs=+-
  Blockout_i_d_SG_D_1_03b31 : Outport
  wires:
  Constant_-1_005d7/1 -> Product_30dc6/1
  Constant_x_l_26c6b/1 -> Product_30dc6/2
  Constant_x_ddd_e1583/1 -> Subtract_cd319/2
  Product_30dc6/1 -> Add_b559d/1
  Constant_x_qdd_134fa/1 -> Subtract_92451/2
  Constant_x_l_b74c1/1 -> Product_8e0a1/2
  Constant_x_qd_b849d/1 -> Add_6e688/2
  Constant_x_qdd_9bdcd/1 -> Add_b559d/2
  Constant_x_qd_e0d58/1 -> Subtract_92451/1
  MathFunc_cos_2d020/1 -> Product_e93c7/2
  Constant_-1_0dfb2/1 -> Product_8e0a1/1
  Constant_-1_e05e3/1 -> Product_b336d/1
  Subtract_45595/1 -> Blockout_i_d_SG_D_1_03b31/1
  Constant_x_l_c7e57/1 -> Product_b336d/2
  Divide_1dc21/1 -> Subtract_d3172/1
  State_psi_gq_SG_D_1_06924/1 -> Product_07601/1
  Subtract_20919/1 -> Product_9d8c5/2
  Add_b559d/1 -> Product_07601/2
  Divide_7b0e4/1 -> Add_2e8b6/1
  Product_8e0a1/1 -> Add_2610a/1
  Constant_x_qd_64ab0/1 -> Add_2610a/2
  State_psi_kq_SG_D_1_04692/1 -> Product_2fce4/1
  Add_2e8b6/1 -> Subtract_c67a9/1
  Add_2610a/1 -> Divide_1dc21/2
  Subtract_92451/1 -> Product_2fce4/2
  Product_b336d/1 -> Add_6e688/1
  Constant_-1_51d10/1 -> Product_4bd24/1
  State_psi_1d_SG_D_1_017fc/1 -> Product_4bd24/2
  Constant_x_dd_bb0c8/1 -> Subtract_cd319/1
  Product_07601/1 -> Divide_1dc21/1
  Product_8023f/1 -> Divide_aec55/1
  Subtract_cd319/1 -> Product_b0550/2
  Product_2fce4/1 -> Divide_4b9cf/1
  Product_4bd24/1 -> Product_b0550/1
  Add_6e688/1 -> Divide_4b9cf/2
  Constant_x_dd_8242f/1 -> Subtract_322c6/1
  Subtract_d3172/1 -> Add_9e60c/1
  Constant_x_l_cb232/1 -> Subtract_322c6/2
  Constant_x_ddd_2a6be/1 -> Subtract_20919/1
  Constant_x_l_cd88d/1 -> Subtract_20919/2
  Divide_aec55/1 -> Subtract_45595/2
  Divide_4b9cf/1 -> Subtract_d3172/2
  State_theta_SG_D_1_ace1c/1 -> MathFunc_cos_2d020/1
  Product_b0550/1 -> Divide_7b0e4/1
  Subtract_322c6/1 -> Divide_7b0e4/2
  State_theta_SG_D_1_7475d/1 -> MathFunc_sin_75e4b/1
  State_psi_fd_SG_D_1_d596f/1 -> Product_9d8c5/1
  Constant_x_dd_b3416/1 -> Subtract_eb230/1
  Constant_x_l_ff016/1 -> Subtract_eb230/2
  State_psi_q_SG_D_1_1a988/1 -> Add_9e60c/2
  State_psi_d_SG_D_1_ee150/1 -> Add_2e8b6/2
  Constant_x_ddd_39085/1 -> Divide_aec55/2
  MathFunc_sin_75e4b/1 -> Product_8023f/2
  Product_9d8c5/1 -> Divide_f4998/1
  Constant_-1_b9eea/1 -> Product_8793c/1
  Subtract_eb230/1 -> Divide_f4998/2
  Add_9e60c/1 -> Product_8793c/2
  Divide_f4998/1 -> Subtract_c67a9/2
  Product_8793c/1 -> Product_e93c7/1
  Subtract_c67a9/1 -> Product_8023f/1
  Constant_x_qdd_f3715/1 -> Divide_15d94/2
  Product_e93c7/1 -> Divide_15d94/1
  Divide_15d94/1 -> Subtract_45595/1

== system case3/SG_D_1/i_q_SG_D_1_block ==
  note: i_q_SG_D_1 in case3
      | $-\frac{\sin\left(\theta _{\mathrm{SG},D,1}\right)\,\left(\psi _{q,\mathrm{SG},D,1}+\frac{\psi _{\mathrm{gq},\mathrm{SG},D,1}\,\left(x_{l}-x_{\mathrm{qdd}}\right)}{x_{l}-x_{\mathrm{qd}}}+\frac{\psi _{\mathrm{kq},\mathrm{SG},D,1}\,\left(x_{\mathrm{qd}}-x_{\mathrm{qdd}}\right)}{x_{l}-x_{\mathrm{qd}}}\right)}{x_{\mathrm{qdd}}}-\frac{\cos\left(\theta _{\mathrm{SG},D,1}\right)\,\left(\frac{\psi _{\mathrm{1d},\mathrm{SG},D,1}\,\left(x_{\mathrm{dd}}-x_{\mathrm{ddd}}\right)}{x_{\mathrm{dd}}-x_{l}}-\psi _{d,\mathrm{SG},D,1}+\frac{\psi _{\mathrm{fd},\mathrm{SG},D,1}\,\left(x_{\mathrm{ddd}}-x_{l}\right)}{x_{\mathrm{dd}}-x_{l}}\right)}{x_{\mathrm{ddd}}}$
      | Automatically generated on 2025-10-31 18:59:34 .
  State_psi_gq_SG_D_1_d01d3 : Inport
  State_psi_kq_SG_D_1_9d437 : Inport  Port=2
  State_psi_q_SG_D_1_8c0e7 : Inport  Port=3
  State_theta_SG_D_1_2faf8 : Inport  Port=4
  State_psi_1d_SG_D_1_0c5a6 : Inport  Port=5
  State_psi_d_SG_D_1_f3b11 : Inport  Port=6
  State_psi_fd_SG_D_1_33a9d : Inport  Port=7
  State_theta_SG_D_1_efa60 : Inport  Port=8
  Add_317f8 : Sum
  Add_3d3ee : Sum
  Add_9771d : Sum
  Add_a5ba6 : Sum
  Add_a8c28 : Sum
  Add_ee68d : Sum
  Constant_-1_06545 : Constant  Value=-1
  Constant_-1_147c9 : Constant  Value=-1
  Constant_-1_46d42 : Constant  Value=-1
  Constant_-1_62af8 : Constant  Value=-1
  Constant_-1_6a189 : Constant  Value=-1
  Constant_x_dd_076ad : Constant  Value=x_dd
  Constant_x_dd_16041 : Constant  Value=x_dd
  Constant_x_dd_ed15b : Constant  Value=x_dd
  Constant_x_ddd_99199 : Constant  Value=x_ddd
  Constant_x_ddd_adcf3 : Constant  Value=x_ddd
  Constant_x_ddd_b2c58 : Constant  Value=x_ddd
  Constant_x_l_193d0 : Constant  Value=x_l
  Constant_x_l_1df59 : Constant  Value=x_l
  Constant_x_l_1f28e : Constant  Value=x_l
  Constant_x_l_5634f : Constant  Value=x_l
  Constant_x_l_c4e3e : Constant  Value=x_l
  Constant_x_l_ebc0a : Constant  Value=x_l
  Constant_x_qd_17ba0 : Constant  Value=x_qd
  Constant_x_qd_30688 : Constant  Value=x_qd
  Constant_x_qd_4e8bb : Constant  Value=x_qd
  Constant_x_qdd_01dc1 : Constant  Value=x_qdd
  Constant_x_qdd_4de0a : Constant  Value=x_qdd
  Constant_x_qdd_b9f09 : Constant  Value=x_qdd
  Divide_02e41 : Product  Inputs=*/
  Divide_2c568 : Product  Inputs=*/
  Divide_318dc : Product  Inputs=*/
  Divide_6caa3 : Product  Inputs=*/
  Divide_8b7bf : Product  Inputs=*/
  Divide_f0f1a : Product  Inputs=*/
  MathFunc_cos_49ea6 : Trigonometry  Operator=cos
  MathFunc_sin_d5418 : Trigonometry
  Product_19ded : Product
  Product_5de87 : Product
  Product_5ee86 : Product
  Product_61221 : Product
  Product_70760 : Product
  Product_80475 : Product
  Product_93df4 : Product
  Product_9438a : Product
  Product_c35e0 : Product
  Product_d95dc : Product
  Product_dec9b : Product
  Subtract_096c6 : Sum  Inputs=+-
  Subtract_157e9 : Sum  Inputs=+-
  Subtract_37219 : Sum  Inputs=+-
  Subtract_4e030 : Sum  Inputs=+-
  Subtract_7822e : Sum  Inputs=+-
  Subtract_8f7fe : Sum  Inputs=+-
  Subtract_a6897 : Sum  Inputs=+-
  Blockout_i_q_SG_D_1_dd5f1 : Outport
  wires:
  State_theta_SG_D_1_efa60/1 -> MathFunc_cos_49ea6/1
  State_psi_fd_SG_D_1_33a9d/1 -> Product_70760/1
  Constant_-1_6a189/1 -> Product_5de87/1
  Constant_x_l_5634f/1 -> Product_5de87/2
  Subtract_8f7fe/1 -> Product_70760/2
  Constant_x_l_1f28e/1 -> Subtract_37219/2
  Product_5de87/1 -> Add_a5ba6/1
  Constant_x_qdd_4de0a/1 -> Add_a5ba6/2
  Constant_x_qd_4e8bb/1 -> Subtract_4e030/1
  Constant_x_qdd_b9f09/1 -> Divide_02e41/2
  MathFunc_sin_d5418/1 -> Product_19ded/2
  Constant_-1_46d42/1 -> Product_c35e0/1
  Constant_x_qdd_01dc1/1 -> Subtract_4e030/2
  Add_9771d/1 -> Product_93df4/2
  Product_5ee86/1 -> Divide_6caa3/1
  Constant_x_l_c4e3e/1 -> Product_c35e0/2
  Constant_-1_147c9/1 -> Product_d95dc/1
  Constant_x_l_1df59/1 -> Product_d95dc/2
  State_psi_gq_SG_D_1_d01d3/1 -> Product_5ee86/1
  Add_a5ba6/1 -> Product_5ee86/2
  Divide_f0f1a/1 -> Add_3d3ee/1
  Product_c35e0/1 -> Add_ee68d/1
  Divide_02e41/1 -> Add_a8c28/1
  Constant_x_qd_17ba0/1 -> Add_ee68d/2
  State_psi_kq_SG_D_1_9d437/1 -> Product_9438a/1
  Add_3d3ee/1 -> Subtract_157e9/1
  Subtract_4e030/1 -> Product_9438a/2
  Divide_6caa3/1 -> Subtract_a6897/1
  Add_ee68d/1 -> Divide_6caa3/2
  Product_d95dc/1 -> Add_317f8/1
  Constant_x_qd_30688/1 -> Add_317f8/2
  Constant_-1_62af8/1 -> Product_61221/1
  MathFunc_cos_49ea6/1 -> Product_80475/2
  Product_70760/1 -> Divide_8b7bf/1
  State_psi_1d_SG_D_1_0c5a6/1 -> Product_61221/2
  Constant_x_l_193d0/1 -> Subtract_7822e/2
  Constant_x_dd_076ad/1 -> Subtract_096c6/1
  Divide_8b7bf/1 -> Subtract_157e9/2
  Constant_x_ddd_adcf3/1 -> Subtract_096c6/2
  Product_80475/1 -> Divide_318dc/1
  Product_9438a/1 -> Divide_2c568/1
  Product_61221/1 -> Product_dec9b/1
  Add_317f8/1 -> Divide_2c568/2
  Subtract_096c6/1 -> Product_dec9b/2
  State_psi_d_SG_D_1_f3b11/1 -> Add_3d3ee/2
  Constant_x_dd_ed15b/1 -> Subtract_37219/1
  Constant_x_ddd_b2c58/1 -> Subtract_8f7fe/1
  Constant_x_l_ebc0a/1 -> Subtract_8f7fe/2
  Divide_318dc/1 -> Add_a8c28/2
  Divide_2c568/1 -> Subtract_a6897/2
  State_theta_SG_D_1_2faf8/1 -> MathFunc_sin_d5418/1
  Product_dec9b/1 -> Divide_f0f1a/1
  Subtract_37219/1 -> Divide_f0f1a/2
  Constant_x_dd_16041/1 -> Subtract_7822e/1
  Subtract_a6897/1 -> Add_9771d/1
  State_psi_q_SG_D_1_8c0e7/1 -> Add_9771d/2
  Subtract_7822e/1 -> Divide_8b7bf/2
  Subtract_157e9/1 -> Product_80475/1
  Constant_-1_06545/1 -> Product_93df4/1
  Product_93df4/1 -> Product_19ded/1
  Product_19ded/1 -> Divide_02e41/1
  Constant_x_ddd_99199/1 -> Divide_318dc/2
  Add_a8c28/1 -> Blockout_i_q_SG_D_1_dd5f1/1

== system case3/SG_D_1/theta_SG_D_1_out_block ==
  note: theta_SG_D_1_out in case3
      | $\theta _{\mathrm{SG},D,1}$
      | Automatically generated on 2025-10-31 18:59:39 .
  State_theta_SG_D_1_c9680 : Inport
  Blockout_theta_SG_D_1_out_2820c : Outport
  wires:
  State_theta_SG_D_1_c9680/1 -> Blockout_theta_SG_D_1_out_2820c/1

== system case3/SG_D_1/w_SG_D_1_out_block ==
  note: w_SG_D_1_out in case3
      | $w_{\mathrm{SG},D,1}$
      | Automatically generated on 2025-10-31 18:59:39 .
  State_w_SG_D_1_fc530 : Inport
  Blockout_w_SG_D_1_out_d9996 : Outport
  wires:
  State_w_SG_D_1_fc530/1 -> Blockout_w_SG_D_1_out_d9996/1
